simulink model "simulink_projesi"  (R2019a)
settings: Solver=VariableStepAuto  StartTime=0.0  StopTime=10.0  RelTol=1e-3
settings Model: Creator=PC_393_ADMIN  LastModifiedBy=PC_566_ADMIN

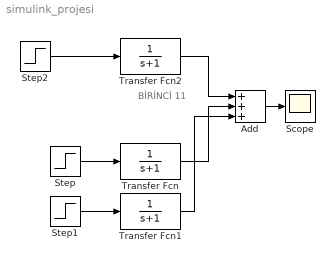
== system simulink_projesi ==
  note: BİRİNCİ 11
  Add : Sum  Inputs=+++
  Scope : Scope
  Step : Step  SampleTime=0
  Step1 : Step  SampleTime=0
  Step2 : Step  SampleTime=0
  Transfer Fcn : TransferFcn  Denominator=[1 1]
  Transfer Fcn1 : TransferFcn  Denominator=[1 1]
  Transfer Fcn2 : TransferFcn  Denominator=[1 1]
  wires:
  Transfer Fcn/1 -> Add/2
  Step/1 -> Transfer Fcn/1
  Step1/1 -> Transfer Fcn1/1
  Transfer Fcn2/1 -> Add/1
  Step2/1 -> Transfer Fcn2/1
  Add/1 -> Scope/1
  Transfer Fcn1/1 -> Add/3
